simulink model "Model"  (R2021a)
settings: Solver=FixedStepDiscrete  StartTime=0.0  StopTime=inf  RelTol=1e-3
model workspace (MAT data in the model file):
  F0 = 44100
libraries: audiosources x2, dspsnks4 x1, dspfdesign x1
settings Model: Creator=Kazuki Matsumoto  LastModifiedBy=Kazuki Matsumoto
settings SolverCC: AlgebraicLoopSolver=TrustRegion  AutoInsertRateTranBlk=on
settings DataIOCC: LimitDataPoints=on  SaveOutput=off  SignalLogging=off  SaveTime=off
settings OptimizationCC: LifeSpan=inf
settings DebuggingCC: AlgebraicLoopMsg=error  SingleTaskRateTransMsg=error  AllowSymbolicDim=off  SFUnexpectedBacktrackingDiag=warning  SFNoUnconditionalDefaultTransitionDiag=warning  SFExecutionAtInitializationDiag=none  SFMachineParentedDataDiag=warning  ArithmeticOperatorsInVariantConditions=warning
settings SFSimCC: SimUseLocalCustomCode=off  CustomCodeUndefinedFunction=UseInterfaceOnly
settings RTWCC: RTWUseLocalCustomCode=off
settings CodeAppCC: StateflowObjectComments=on
settings GRTTargetCC: TargetLangStandard=C89/C90 (ANSI)
settings ConfigComp: CovMetricSettings=dw  CovSaveCumulativeToWorkspaceVar=on  CovSaveSingleToWorkspaceVar=on  CovExternalEMLEnable=off  CovSFcnEnable=off

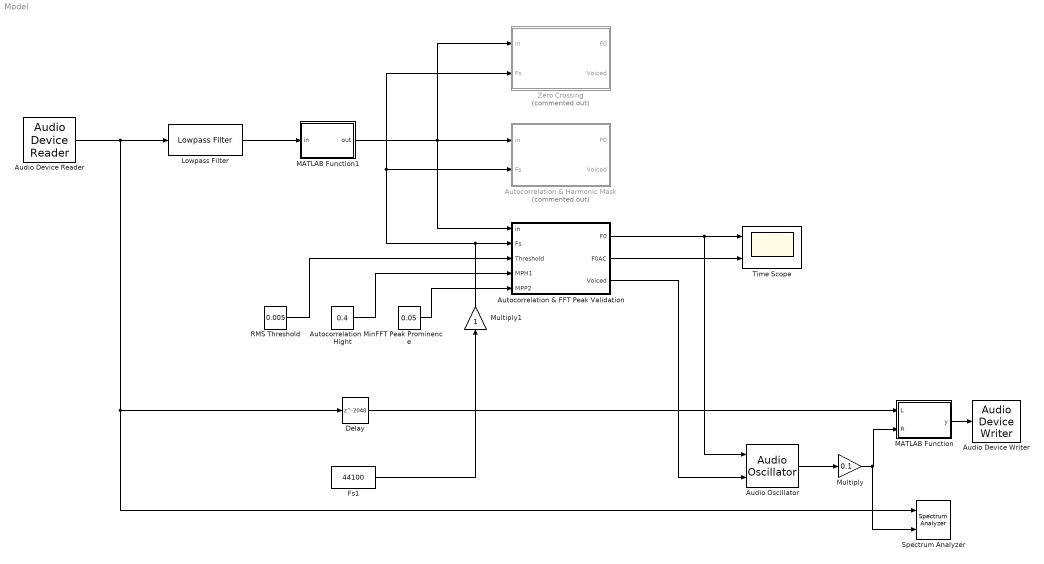
== system Model ==
  Audio Device Reader : audiosources/Audio Device Reader  Driver=DirectSound  Device=ライン (Steinberg UR12 )  SampleRate=44100  NumChannels=1  SamplesPerFrame=1024  BitDepth=16-bit integer  NumBuffers=10  DefaultInputChannelMapping=on  InputChannelMapping=1:2  OutputNumOverrunSamples=off  OutputDataType=double  DriverIdx=1  DeviceWarnFlag=''
      settings: SourceProductBaseCode=AU
  Audio Device Writer : dspsnks4/Audio Device Writer  Driver=DirectSound  Device=Default  InheritSampleRate=on  SampleRate=8000  BitDepth=16-bit integer  BufferSize=4096  NumBuffers=10  DefaultOutputChannelMapping=on  OutputChannelMapping=1:2  OutputNumUnderrunSamples=off  DriverIdx=1  DeviceWarnFlag=''
  Audio Oscillator : audiosources/Audio Oscillator  FrequencyPort=on  Frequency=100  AmplitudePort=on  Amplitude=0.3  DCOffsetPort=off  PhaseOffset=0  DCOffset=0  WidthPort=off  Width=1  DutyCyclePort=off  DutyCycle=0.5  SampsPerFrame=1024  Fs=44100  OutputDataType=double  SimulateUsing=Code generation
      settings: SourceProductBaseCode=AU  SignalType=sawtooth
  Autocorrelation Min Hight : Constant  Value=0.4
  Autocorrelation & FFT Peak Validation : MATLAB Function  TreatAsAtomicUnit=on
  Autocorrelation & Harmonic Mask : MATLAB Function  Commented=on  TreatAsAtomicUnit=on
  Delay : Delay  DelayLength=2048  InitialCondition=0  InputProcessing=Columns as channels (frame based)  UseCircularBuffer=on
  FFT Peak Prominence : Constant  Value=0.05
  Fs1 : Constant  Value=44100
  Lowpass Filter : dspfdesign/Lowpass Filter  FilterType=FIR  DesignForMinimumOrder=on  FilterOrder=50  PassbandFrequency=5e1  StopbandFrequency=2e3  PassbandRipple=0.1  StopbandAttenuation=80  InheritSampleRate=off  SampleRate=44100  SimulateUsing=Interpreted execution  roundingMode=Floor  coeffsDataTypeStr=fixdt(1,16)
  MATLAB Function : MATLAB Function  TreatAsAtomicUnit=on
  MATLAB Function1 : MATLAB Function  TreatAsAtomicUnit=on
  Multiply : Gain  Gain=0.1
  Multiply1 : Gain
  RMS Threshold : Constant  Value=0.005
  Spectrum Analyzer : SpectrumAnalyzer  NumInputPorts=2
  Time Scope : Scope  NumInputPorts=2
  Zero Crossing : MATLAB Function  Commented=on  TreatAsAtomicUnit=on
  wires:
  Multiply1/1 -> Zero Crossing/2(Fs), Autocorrelation & Harmonic Mask/2(Fs), Autocorrelation & FFT Peak Validation/2(Fs)
  Audio Oscillator/1 -> Multiply/1
  Lowpass Filter/1 -> MATLAB Function1/1(in)
  Fs1/1 -> Multiply1/1
  Delay/1 -> MATLAB Function/1(L)
  MATLAB Function/1(y) -> Audio Device Writer/1
  Multiply/1 -> Spectrum Analyzer/2, MATLAB Function/2(R)
  RMS Threshold/1 -> Autocorrelation & FFT Peak Validation/3(Threshold)
  Autocorrelation Min Hight/1 -> Autocorrelation & FFT Peak Validation/4(MPH1)
  FFT Peak Prominence/1 -> Autocorrelation & FFT Peak Validation/5(MPP2)
  Autocorrelation & FFT Peak Validation/3(Voiced) -> Audio Oscillator/2
  Audio Device Reader/1 -> Spectrum Analyzer/1, Delay/1, Lowpass Filter/1
  Autocorrelation & FFT Peak Validation/1(F0) -> Audio Oscillator/1, Time Scope/1
  Autocorrelation & FFT Peak Validation/2(F0AC) -> Time Scope/2
  MATLAB Function1/1(out) -> Zero Crossing/1(in), Autocorrelation & FFT Peak Validation/1(in), Autocorrelation & Harmonic Mask/1(in)

== matlab function Model/MATLAB Function1 ==
  data: in input; out output
function out = fcn(in)
    in = flipud(in);

    N = 4096;

    persistent Buffer
    if isempty(Buffer)
        Buffer = zeros(N,1);
    end
    
    if length(in) < N
        Buffer(length(in)+1:end) = Buffer(1:end-length(in));
        Buffer(1:length(in))= in(1:length(in));
    else
        Buffer = in(1:N);
    end
    
    %{
    clf;
    plot(Buffer);
    drawnow;
    %}
    
    out = Buffer;

== matlab function Model/Zero Crossing ==
  data: in input; Fs input; F0 output; Voiced output
function [F0, Voiced] = fcn(in,Fs)

    in = in;

    persistent f
    if isempty(f)
        f = figure(1);
    end
    
    rmsvalue = rms(in);
    calc_diff = @(X) [X(1);X].*[X;X(end)];
    cross = find(calc_diff(in) < 0);
    if length(cross) > 3 && rmsvalue > 0.01
        T = cross(3:end)-cross(1:end-2);
        F0 = Fs/mean(T);
        Voiced = 1;
    else
        F0 = 0;
        Voiced = 0;
    end
    
    %{
    clf;
    title("F0 Estimation (Zero Crossing)");
    subplot(2,1,1);
    hold on;title("Waveform")
    plot(in,Color="r");xlim([-inf inf]);ylim([-0.5,0.5]);
    plot([0,length(in)],[0,0],Color="k");
    plot([0,length(in)],[rmsvalue,rmsvalue],Color="b");
    plot(cross,zeros(size(cross)),"o",Color = "red");
    xlabel("Sample");ylabel("Amptitude");
    %}
end

== matlab function Model/Autocorrelation & Harmonic Mask ==
  data: in input; Fs input; F0 output; Voiced output
function [F0, Voiced] = fcn(in,Fs)
    
    %% Init
    coder.extrinsic("imagesc");
    coder.extrinsic("xline");
    coder.extrinsic("legend");
    coder.extrinsic("bar");
    coder.extrinsic("area");
    
    persistent f
    persistent F0Buff
    persistent F0ACBuff
    persistent SBuff
    persistent WinFunc
    
    BuffN = 50;
    
    if isempty(f)
        f = figure(1);
        F0Buff = zeros(1,BuffN);
        F0ACBuff = zeros(1,BuffN);
        SBuff  = zeros(length(in)/2,BuffN);
        WinFunc = blackman(length(in));
    end
    
    %% Estimate F0
    
    rmsvalue = rms(in);
    
    AC = xcorr(in);
    AC = AC(floor(end/2):end);
    AC = AC/AC(1);
    
    clf;
    title("F0 Estimation (Zero Crossing)");
    
    subplot(2,3,1);
    hold on;title("Autocorrection");
    
    [~,locs] = findpeaks(AC);
    if rmsvalue > 0.01 && length(locs) >= 2
        plot(locs,AC(locs),"o",color="r")
        F0 = 1/mean(locs(2:end)-locs(1:end-1))*Fs;
        Voiced = 1;
    else
        F0 = 0;
        Voiced = 0;
    end
    
    plot(AC,color="k");
    xlim([-inf inf]);ylim([-1 1]);
    grid off;    
    xlabel("sample");ylabel("Amptitude");
    
    %% Correct F0
    
    preemph = [1 -0.97];
    S = abs(fft(filter(preemph,1,in).*WinFunc));
    S = S(1:end/2);
    
    function mask = harmonic_mask(F0,Fs,N,nfft)
        mask = zeros(nfft/2,1);
        for i = 1:5
            F0idx = floor(nfft*F0/N*i/(Fs)+0.5)+1;
            mask(max(F0idx,1)) = 1;
        end
    end

    M1     = harmonic_mask(F0,Fs,1,length(in));
    M2     = harmonic_mask(F0,Fs,2,length(in));
    M3     = harmonic_mask(F0,Fs,3,length(in));
    
    Smax = max(S);
    
    L1 = sum(S.*M1/Smax);
    L2 = sum(S.*M2/Smax);
    L3 = sum(S.*M3/Smax);
    
    L = [L1 L2 L3]*Voiced;
    [~,maxL] = max(L);
    
    F0AC = F0;
    F0 = F0 / maxL;
    
    subplot(2,3,2);hold on;
    title("fft");
    freq = linspace(0,Fs/2,length(in)/2);
    plot(freq,S/Smax);plot(freq,M1);plot(freq,M2);plot(freq,M3);
    xlim([-inf inf]);ylim([0,1.1]);
    xline(F0);
    set(gca,'XScale','log')
    
    subplot(2,3,3);
    bar(L);
    ylim([0,10]);
    title("Normalized Likelihood")
    
    %% F0 Plot
    F0Buff = [F0, F0Buff(1:end-1)];
    F0ACBuff = [F0AC, F0ACBuff(1:end-1)];
    SBuff = [S, SBuff(:,1:end-1)];
    freq  = linspace(1,Fs/2,length(in));
    
    subplot(2,1,2);
    title("F0");
    hold on;
    colormap("gray");imagesc(1:BuffN,freq,log(fliplr(SBuff)));
    semilogy(fliplr(F0ACBuff),".",Color="blue");
    semilogy(fliplr(F0Buff),".",Color="red");
    xlim([1 length(F0Buff)]);ylim([0,2000]);
    xlabel("Frame");ylabel("Frequency");
    legend("F0","F0 (Corrected)")
    drawnow;
end

== matlab function Model/MATLAB Function ==
  data: L input; y output; R input
function y = fcn(L, R)
coeff = 1;
y = [coeff*L+R, L+coeff*R]/(coeff+1);
end

== matlab function Model/Autocorrelation & FFT Peak Validation ==
  data: in input; Fs input; Threshold input; MPH1 input; F0 output; F0AC output; Voiced output; MPP2 input
function [F0, F0AC, Voiced] = fcn(in,Fs,Threshold,MPH1,MPP2)
    
    %% Init
    coder.extrinsic("imagesc");
    coder.extrinsic("xline");
    coder.extrinsic("yline");
    coder.extrinsic("legend");
    coder.extrinsic("bar");
    coder.extrinsic("area");
    
    persistent f
    persistent F0Buff
    persistent F0ACBuff
    persistent SBuff
    persistent WinFunc
    persistent WinFunc2
    
    BuffN = 50;
    
    if isempty(f)
        f = figure(1);
        F0Buff = zeros(1,BuffN);
        F0ACBuff = zeros(1,BuffN);
        SBuff  = zeros(length(in)/2,BuffN);
        WinFunc = blackman(length(in));
        WinFunc2 = blackman(length(in)*2);
    end
    
    %% Estimate F0
    
    F0min = 80;
    
    rmsvalue = rms(in);
    
    AC = xcorr(in);
    AC = AC(floor(end/2):end);
    
    AClen = length(AC);
    AC = AC(1:end-1)./fliplr(1:AClen-1)';
    AC = AC/AC(1);
    
    [~,locsAC] = findpeaks(AC,'MinPeakHeight',MPH1);
    
    if rmsvalue > Threshold && ...
            length(locsAC) >= 2 ...
            
        % Diff
        D = locsAC(2:end)-locsAC(1:end-1);
        
        % Check the First Peak
        F0 = 1/D(1)*Fs;
        if F0 < F0min
            Voiced = 0;
        else
            W = round(D/D(1));
            W(W>=3) = 0;

            F0 = 1/(sum(D.*W)./sum(W))*Fs;
            Voiced = 1;
        end
        
    else
        F0 = 0;
        Voiced = 0;
    end
    
    %% Correct F0
    
    F0AC = F0;
    
    preemph = [1, -0.96];
    S = abs(fft(filter(preemph,1,in).*WinFunc));
    Smax = max(S);
    S = S(1:end/2)/Smax;
    
    [~,locsFFT] = findpeaks(S,'MinPeakProminence',MPP2);
    
    % Check the F0 range
    if F0 < F0min
        Voiced = 0;
        F0 = 0;
    end
    
    % Convert F0 to Index
    F0idx = length(in)*F0/Fs+1;
    
    % Check F0/2;
    if ( any(floor(F0idx/2)-1 <= locsFFT)  &&...
         any(locsFFT <= floor(F0idx/2)+1)) &&...
         F0min <= F0/2
        
        F0 = F0/2;
    end
    
    %% Plot
    %%{
    clf;
    title("F0 Estimation (Zero Crossing)");
    
    subplot(2,2,1);
    hold on;title("Autocorrection /(N - Sample)");
    
    if Voiced
        plot(locsAC,AC(locsAC),"o",color="r")
    end
    plot(AC,color="k");plot(WinFunc2(end/2+1:end),color="b")
    yline(MPH1)
    xlim([-inf inf]);ylim([-1.1 1.1]);
    grid off;
    xlabel("sample");ylabel("Amptitude");
    
    freq = linspace(0,Fs/2,length(in)/2);
    subplot(2,2,2);hold on;
    
    if Voiced
        plot(freq(locsFFT),S(locsFFT),"o",color="r")
        xline(F0);
    end
    
    title("fft");
    plot(freq,S,"color","k");
    xlim([-inf inf]);ylim([0,1.1]);
    set(gca,'XScale','log')
    
    F0Buff = [F0, F0Buff(1:end-1)];
    F0ACBuff = [F0AC, F0ACBuff(1:end-1)];
    SBuff = [S, SBuff(:,1:end-1)];
    freq  = linspace(1,Fs/2,length(in));
    
    subplot(2,1,2);
    title("F0");
    hold on;
    colormap("gray");imagesc(1:BuffN,freq,log(fliplr(SBuff)));
    semilogy(fliplr(F0ACBuff),".--",Color="blue");
    semilogy(fliplr(F0Buff),".--",Color="red");
    xlim([1 length(F0Buff)]);ylim([0,2000]);
    xlabel("Frame");ylabel("Frequency");
    legend("F0","F0 (Corrected)")
    drawnow;
    %}
end
